simulink model "21-E"  (R2014a)
settings: Solver=FixedStepDiscrete  StartTime=0.0  StopTime=10.0  FixedStep=0.0005  RelTol=1e-3
undefined symbols (not defined in the file): add_k1_100, add_k2_100, ADDspeed, cal_acc_div, cal_acc_flo_add, cal_acc_min, cal_an_div, cal_an_min, cal_bre_div, cal_bre_en_add, cal_bre_flo_add, cal_bre_min, cal_conf_off, cal_conf_on, controller, ecucoder_acal, enres_on_add, enres_per_add
libraries: simulink x165, ec55xxlib x29
(part 1 of 6)
settings Model: Creator=ASUS  LastModifiedBy=ASUS
settings OptimizationCC: InlineParams=on  InlineInvariantSignals=on  RollThreshold=9  StateBitsets=on  DataBitsets=on  UseTempVars=on  ZeroExternalMemoryAtStartup=off  ZeroInternalMemoryAtStartup=off  EfficientFloat2IntCast=on  OptimizeModelRefInitCode=on  LifeSpan=1
settings DebuggingCC: InheritedTsInSrcMsg=none
settings HardwareCC: ProdLargestAtomicInteger=Long  ProdLargestAtomicFloat=Double  ProdIntDivRoundTo=Zero  ProdEndianess=BigEndian  ProdHWDeviceType=Freescale MPC5500
settings RTWCC: SystemTargetFile=ec55xx.tlc  MakeCommand=make_rtw optimized_fixed_point=1  GenerateMakefile=off  TemplateMakefile=ec55xx_lcc.tmf  PostCodeGenCommand=ec55xx_pst_s2(buildInfo)  Description=Target for EC55XX  GenerateReport=on  ProcessScript=ec55xx_make_rtw_hook  IncludeHyperlinkInReport=on  LaunchReport=on
settings CodeAppCC: IgnoreCustomStorageClasses=off
settings STFCustomTargetCC: ModelReferenceCompliant=off  ConcurrentExecutionCompliant=off  IncludeMdlTerminateFcn=off  GeneratePreprocessorConditionals=Use local settings  CombineOutputUpdateFcns=on  SuppressErrorStatus=on  ERTCustomFileBanners=on  SupportContinuousTime=off  SupportNonInlinedSFcns=off  MATLABClassNameForMDSCustomization=Simulink.SoftwareTarget.ERTCustomization  GRTInterface=off  SystemTargetFile=ec55xx.tlc
settings ERTTargetCC: GenerateSampleERTMain=off  ModelReferenceCompliant=off  IncludeMdlTerminateFcn=off  SuppressErrorStatus=on  GenerateASAP2=on  ERTSrcFileBannerTemplate=ec55xx_code_template.cgt  ERTHdrFileBannerTemplate=ec55xx_code_template.cgt  ERTDataSrcFileTemplate=ec55xx_code_template.cgt  ERTDataHdrFileTemplate=ec55xx_code_template.cgt  ERTCustomFileTemplate=ec55xx_file_process.tlc

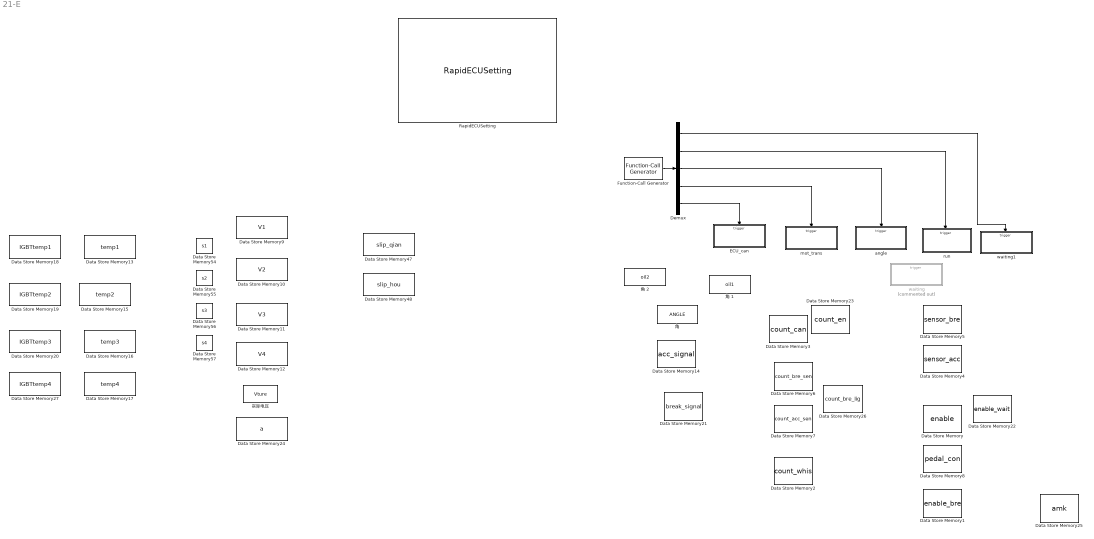
== system 21-E ==
  Data Store Memory : DataStoreMemory  DataStoreName=enable  ReadBeforeWriteMsg=warning  WriteAfterWriteMsg=warning  WriteAfterReadMsg=warning  OutDataTypeStr=boolean
  Data Store Memory1 : DataStoreMemory  DataStoreName=enable_bre  ReadBeforeWriteMsg=warning  WriteAfterWriteMsg=warning  WriteAfterReadMsg=warning  OutDataTypeStr=boolean
  Data Store Memory10 : DataStoreMemory  DataStoreName=V2  ReadBeforeWriteMsg=warning  WriteAfterWriteMsg=warning  WriteAfterReadMsg=warning  OutMin=-13000  OutMax=13000  OutDataTypeStr=double
  Data Store Memory11 : DataStoreMemory  DataStoreName=V3  ReadBeforeWriteMsg=warning  WriteAfterWriteMsg=warning  WriteAfterReadMsg=warning  OutMin=-13000  OutMax=13000  OutDataTypeStr=double
  Data Store Memory12 : DataStoreMemory  DataStoreName=V4  ReadBeforeWriteMsg=warning  WriteAfterWriteMsg=warning  WriteAfterReadMsg=warning  OutMin=-13000  OutMax=13000  OutDataTypeStr=double
  Data Store Memory13 : DataStoreMemory  DataStoreName=temp1  ReadBeforeWriteMsg=warning  WriteAfterWriteMsg=warning  WriteAfterReadMsg=warning  OutDataTypeStr=int16
  Data Store Memory14 : DataStoreMemory  DataStoreName=acc_signal  ReadBeforeWriteMsg=warning  WriteAfterWriteMsg=warning  WriteAfterReadMsg=warning  OutDataTypeStr=double
  Data Store Memory15 : DataStoreMemory  DataStoreName=temp2  ReadBeforeWriteMsg=warning  WriteAfterWriteMsg=warning  WriteAfterReadMsg=warning  OutDataTypeStr=int16
  Data Store Memory16 : DataStoreMemory  DataStoreName=temp3  ReadBeforeWriteMsg=warning  WriteAfterWriteMsg=warning  WriteAfterReadMsg=warning  OutDataTypeStr=int16
  Data Store Memory17 : DataStoreMemory  DataStoreName=temp4  ReadBeforeWriteMsg=warning  WriteAfterWriteMsg=warning  WriteAfterReadMsg=warning  OutDataTypeStr=int16
  Data Store Memory18 : DataStoreMemory  DataStoreName=IGBTtemp1  ReadBeforeWriteMsg=warning  WriteAfterWriteMsg=warning  WriteAfterReadMsg=warning  OutDataTypeStr=int16
  Data Store Memory19 : DataStoreMemory  DataStoreName=IGBTtemp2  ReadBeforeWriteMsg=warning  WriteAfterWriteMsg=warning  WriteAfterReadMsg=warning  OutDataTypeStr=int16
  Data Store Memory2 : DataStoreMemory  DataStoreName=count_whis  ReadBeforeWriteMsg=warning  WriteAfterWriteMsg=warning  WriteAfterReadMsg=warning  OutDataTypeStr=double
  Data Store Memory20 : DataStoreMemory  DataStoreName=IGBTtemp3  ReadBeforeWriteMsg=warning  WriteAfterWriteMsg=warning  WriteAfterReadMsg=warning  OutDataTypeStr=int16
  Data Store Memory21 : DataStoreMemory  DataStoreName=break_signal  ReadBeforeWriteMsg=warning  WriteAfterWriteMsg=warning  WriteAfterReadMsg=warning  OutDataTypeStr=double
  Data Store Memory22 : DataStoreMemory  DataStoreName=enable_wait  ReadBeforeWriteMsg=warning  WriteAfterWriteMsg=warning  WriteAfterReadMsg=warning  OutDataTypeStr=boolean
  Data Store Memory23 : DataStoreMemory  DataStoreName=count_en  ReadBeforeWriteMsg=warning  WriteAfterWriteMsg=warning  WriteAfterReadMsg=warning  OutDataTypeStr=double
  Data Store Memory24 : DataStoreMemory  DataStoreName=a  ReadBeforeWriteMsg=warning  WriteAfterWriteMsg=warning  WriteAfterReadMsg=warning  OutMin=-13000  OutMax=13000  OutDataTypeStr=double
  Data Store Memory25 : DataStoreMemory  DataStoreName=amk  ReadBeforeWriteMsg=warning  WriteAfterWriteMsg=warning  WriteAfterReadMsg=warning  OutDataTypeStr=uint16
  Data Store Memory26 : DataStoreMemory  DataStoreName=count_bre_lig  ReadBeforeWriteMsg=warning  WriteAfterWriteMsg=warning  WriteAfterReadMsg=warning  OutDataTypeStr=double
  Data Store Memory27 : DataStoreMemory  DataStoreName=IGBTtemp4  ReadBeforeWriteMsg=warning  WriteAfterWriteMsg=warning  WriteAfterReadMsg=warning  OutDataTypeStr=int16
  Data Store Memory3 : DataStoreMemory  DataStoreName=count_can  ReadBeforeWriteMsg=warning  WriteAfterWriteMsg=warning  WriteAfterReadMsg=warning  OutDataTypeStr=double
  Data Store Memory4 : DataStoreMemory  DataStoreName=sensor_acc  ReadBeforeWriteMsg=warning  WriteAfterWriteMsg=warning  WriteAfterReadMsg=warning  OutDataTypeStr=boolean
  Data Store Memory47 : DataStoreMemory  DataStoreName=slip_qian  ReadBeforeWriteMsg=warning  WriteAfterWriteMsg=warning  WriteAfterReadMsg=warning  OutMin=0  OutMax=1  OutDataTypeStr=double
  Data Store Memory48 : DataStoreMemory  DataStoreName=slip_hou  ReadBeforeWriteMsg=warning  WriteAfterWriteMsg=warning  WriteAfterReadMsg=warning  OutMin=0  OutMax=1  OutDataTypeStr=double
  Data Store Memory5 : DataStoreMemory  DataStoreName=sensor_bre  ReadBeforeWriteMsg=warning  WriteAfterWriteMsg=warning  WriteAfterReadMsg=warning  OutDataTypeStr=boolean
  Data Store Memory54 : DataStoreMemory  DataStoreName=s1  ReadBeforeWriteMsg=warning  WriteAfterWriteMsg=warning  WriteAfterReadMsg=warning  InitialValue=1  OutDataTypeStr=uint16
  Data Store Memory55 : DataStoreMemory  DataStoreName=s2  ReadBeforeWriteMsg=warning  WriteAfterWriteMsg=warning  WriteAfterReadMsg=warning  InitialValue=1  OutDataTypeStr=uint16
  Data Store Memory56 : DataStoreMemory  DataStoreName=s3  ReadBeforeWriteMsg=warning  WriteAfterWriteMsg=warning  WriteAfterReadMsg=warning  InitialValue=1  OutDataTypeStr=uint16
  Data Store Memory57 : DataStoreMemory  DataStoreName=s4  ReadBeforeWriteMsg=warning  WriteAfterWriteMsg=warning  WriteAfterReadMsg=warning  InitialValue=1  OutDataTypeStr=uint16
  Data Store Memory6 : DataStoreMemory  DataStoreName=count_bre_sen  ReadBeforeWriteMsg=warning  WriteAfterWriteMsg=warning  WriteAfterReadMsg=warning  OutDataTypeStr=double
  Data Store Memory7 : DataStoreMemory  DataStoreName=count_acc_sen  ReadBeforeWriteMsg=warning  WriteAfterWriteMsg=warning  WriteAfterReadMsg=warning  OutDataTypeStr=double
  Data Store Memory8 : DataStoreMemory  DataStoreName=pedal_con  ReadBeforeWriteMsg=warning  WriteAfterWriteMsg=warning  WriteAfterReadMsg=warning  OutDataTypeStr=boolean
  Data Store Memory9 : DataStoreMemory  DataStoreName=V1  ReadBeforeWriteMsg=warning  WriteAfterWriteMsg=warning  WriteAfterReadMsg=warning  OutMin=-13000  OutMax=13000  OutDataTypeStr=double
  Demux : Demux  Outputs=5
  ECU_can : Subsystem  TreatAsAtomicUnit=on
  Function-Call Generator : simulink/Ports & Subsystems/Function-Call Generator  sample_time=0.01  numberOfIterations=1
  RapidECUSetting : ec55xxlib/RapidECU_U1/RapidECUSetting
  angle : Subsystem  TreatAsAtomicUnit=on
  mot_trans : Subsystem  TreatAsAtomicUnit=on
  run : Subsystem
  waiting : Subsystem  Commented=on
  waiting1 : Subsystem
  实际电压 : DataStoreMemory  DataStoreName=Vture  ReadBeforeWriteMsg=warning  WriteAfterWriteMsg=warning  WriteAfterReadMsg=warning  OutMin=-13000  OutMax=13000  OutDataTypeStr=double
  "角 " : DataStoreMemory  DataStoreName=ANGLE  ReadBeforeWriteMsg=warning  WriteAfterWriteMsg=warning  WriteAfterReadMsg=warning  OutMin=0  OutMax=1  OutDataTypeStr=double
  角 1 : DataStoreMemory  DataStoreName=oil1  ReadBeforeWriteMsg=warning  WriteAfterWriteMsg=warning  WriteAfterReadMsg=warning  OutMin=0  OutMax=1  OutDataTypeStr=double
  角 2 : DataStoreMemory  DataStoreName=oil2  ReadBeforeWriteMsg=warning  WriteAfterWriteMsg=warning  WriteAfterReadMsg=warning  OutMin=0  OutMax=1  OutDataTypeStr=double
  wires:
  Function-Call Generator/1 -> Demux/1
  Demux/2 -> run/Trigger
  Demux/3 -> angle/Trigger
  Demux/4 -> mot_trans/Trigger
  Demux/1 -> waiting1/Trigger
  Demux/5 -> ECU_can/Trigger

== system 21-E/ECU_can ==
  note: 发送：八个温度
  note: 发送：四轮速
  note: 发送：加速线，加速角，制动油压，制动线，理想和真实侧摆速度，前轮转角，
  note: 发送：滑移率，真实和最大加速度，真实速度，
  Trigger : TriggerPort  TriggerType=function-call  PortDimensions=1
  CANTransmit1 : ec55xxlib/RapidECU_U2/07CANCommucation/CANTransmit  canmodule=B  canbuffer=8  canmessageid=hex2dec('06')  canmessagetype=Standard(11-bit ID)  datalength=8  sampletime=-1
  CANTransmit2 : ec55xxlib/RapidECU_U2/07CANCommucation/CANTransmit  canmodule=B  canbuffer=13  canmessageid=hex2dec('07')  canmessagetype=Standard(11-bit ID)  datalength=8  sampletime=-1
  CAN传输1 : ec55xxlib/RapidECU_U2/07CANCommucation/CANTransmit  canmodule=B  canbuffer=56  canmessageid=hex2dec('05')  canmessagetype=Standard(11-bit ID)  datalength=8  sampletime=-1
  CAN传输4 : ec55xxlib/RapidECU_U2/07CANCommucation/CANTransmit  canmodule=B  canbuffer=15  canmessageid=hex2dec('08')  canmessagetype=Standard(11-bit ID)  datalength=8  sampletime=-1
  Constant{2,4..9} (7 alike) : Constant  Value=100
  Data Store Read : DataStoreRead  DataStoreName=V1
  Data Store Read1 : DataStoreRead  DataStoreName=Vture
  Data Store Read10 : DataStoreRead  DataStoreName=s1
  Data Store Read11 : DataStoreRead  DataStoreName=s2
  Data Store Read12 : DataStoreRead  DataStoreName=s3
  Data Store Read13 : DataStoreRead  DataStoreName=s4
  Data Store Read14 : DataStoreRead  DataStoreName=oil1
  Data Store Read15 : DataStoreRead  DataStoreName=oil2
  Data Store Read2 : DataStoreRead  DataStoreName=ANGLE
  Data Store Read3 : DataStoreRead  DataStoreName=V2
  Data Store Read4 : DataStoreRead  DataStoreName=V3
  Data Store Read5 : DataStoreRead  DialogController=Simulink.DDGSource  DataStoreName=acc_signal
  Data Store Read6 : DataStoreRead  DataStoreName=break_signal
  Data Store Read7 : DataStoreRead  DataStoreName=V4
  Data Store Read8 : DataStoreRead  DataStoreName=slip_qian
  Data Store Read9 : DataStoreRead  DataStoreName=slip_hou
  ECU_dyn1 : Subsystem
  ECU_sig1 : Subsystem
  ECU_speed : Subsystem
  ECU_tem : Subsystem
  Gain : Gain  Gain=1e-6
  Gain1 : Gain  Gain=1e-6
  Product{,1..3} (4 alike) : Product
  Rounding Function{,1..7} (8 alike) : Rounding
  Subsystem : Subsystem
  send1_Ter{,3..5} (4 alike) : Terminator
  wires:
  ECU_tem/1(output) -> CANTransmit1/1
  Subsystem/1(tem4) -> ECU_tem/1(Mot_4_in)
  Subsystem/2(tem3) -> ECU_tem/2(Mot_3_in)
  Subsystem/3(tem2) -> ECU_tem/3(Mot_2_in)
  Subsystem/4(tem1) -> ECU_tem/4(Mot_1_in)
  Subsystem/5(IG4) -> ECU_tem/5(IGBT_4_in)
  Subsystem/6(IG3) -> ECU_tem/6(IGBT_3_in)
  Subsystem/7(IG2) -> ECU_tem/7(IGBT_2_in)
  Subsystem/8(IG1) -> ECU_tem/8(IGBT_1_in)
  Constant9/1 -> ECU_sig1/7(yaw_i_in)
  Constant8/1 -> ECU_sig1/6(yaw_r_in)
  Constant7/1 -> ECU_sig1/4(acc_a_in)
  Rounding Function1/1 -> ECU_sig1/3(bre_l_in)
  Rounding Function5/1 -> ECU_dyn1/7(speed_in)
  Rounding Function4/1 -> ECU_dyn1/5(slip_R_in)
  Rounding Function3/1 -> ECU_dyn1/6(slip_F_in)
  Rounding Function2/1 -> ECU_sig1/8(angle_in)
  Data Store Read9/1 -> Product3/2
  Constant4/1 -> Product3/1
  Product3/1 -> Rounding Function4/1
  Product2/1 -> Rounding Function3/1
  Data Store Read8/1 -> Product2/2
  Constant6/1 -> Product2/1
  Data Store Read7/1 -> ECU_speed/1(v_2R_in)
  Data Store Read4/1 -> ECU_speed/2(v_2L_in)
  Data Store Read3/1 -> ECU_speed/3(v_1R_in)
  Data Store Read/1 -> ECU_speed/4(v_1L_in)
  ECU_speed/1(output) -> CANTransmit2/1
  CANTransmit2/1 -> send1_Ter5/1  "SEND_0x07"
  CANTransmit1/1 -> send1_Ter4/1  "SEND_0x06"
  Data Store Read2/1 -> Rounding Function2/1
  Data Store Read5/1 -> Product/2
  Constant2/1 -> Product/1
  Rounding Function/1 -> ECU_sig1/5(acc_l_in)
  Product1/1 -> Rounding Function1/1
  Constant5/1 -> Product1/2
  Data Store Read6/1 -> Product1/1
  Product/1 -> Rounding Function/1
  Data Store Read1/1 -> Rounding Function5/1
  ECU_dyn1/1(output) -> CAN传输4/1
  CAN传输4/1 -> send1_Ter3/1  "SEND_0x08"
  ECU_sig1/1(output) -> CAN传输1/1
  CAN传输1/1 -> send1_Ter/1  "SEND_0x05"
  Data Store Read10/1 -> ECU_dyn1/4(s_1L_in)
  Data Store Read11/1 -> ECU_dyn1/3(s_1R_in)
  Data Store Read12/1 -> ECU_dyn1/2(s_2L_in)
  Data Store Read13/1 -> ECU_dyn1/1(s_2R_in)
  Data Store Read14/1 -> Gain1/1
  Data Store Read15/1 -> Gain/1
  Gain/1 -> Rounding Function7/1
  Gain1/1 -> Rounding Function6/1
  Rounding Function6/1 -> ECU_sig1/2(bre_o_1_in)
  Rounding Function7/1 -> ECU_sig1/1(bre_o_2_in)

== system 21-E/angle ==
  note: 接收：转角,角速度，最大角速度
  note: 接收：转角,角速度，最大角速度
  Trigger : TriggerPort  TriggerType=function-call  PortDimensions=1
  CAN接收1 : ec55xxlib/RapidECU_U2/07CANCommucation/CANReceive  canmodule=B  canbuffer=16  canmessageid=hex2dec('0001')  canmessagetype=Standard(11-bit ID)  datalength=8  sampletime=-1
  Constant : Constant  Value=2780
  Constant1 : Constant  Value=31
  ECCalVar : Constant  InitFcn=ecucoder_acal;  Value=cal_an_min  OutDataTypeStr=Inherit: Inherit via back propagation  SampleTime=-1
  ECCalVar2 : Constant  InitFcn=ecucoder_acal;  Value=cal_an_div  OutDataTypeStr=Inherit: Inherit via back propagation  SampleTime=-1
  Product1 : Product  Inputs=*/
  Sum : Sum  Inputs=|+-
  Sum1 : Sum  Inputs=|++
  Sum2 : Sum  Inputs=|++
  Terminator{,1..7} (8 alike) : Terminator
  angle2 : Subsystem
  模数转换 : DataTypeConversion  OutDataTypeStr=double
  模数转换1 : DataTypeConversion  OutDataTypeStr=double
  "角 " : DataStoreWrite  DataStoreName=ANGLE
  wires:
  Constant/1 -> Sum1/1
  ECCalVar/1 -> Sum1/2
  Sum/1 -> Product1/1  "calan_min"
  Product1/1 -> "角 "/1  "cal_an"
  Constant1/1 -> Sum2/1
  ECCalVar2/1 -> Sum2/2
  angle2/4(angle_2_Out) -> 模数转换/1  "angle01_2"
  angle2/5(angle_1_Out) -> 模数转换1/1  "angle01_1"
  模数转换/1 -> Terminator/1  "an01_2"
  模数转换1/1 -> Terminator1/1  "an01_1"
  angle2/3(un_1_Out) -> Terminator4/1
  angle2/2(un_2_Out) -> Terminator3/1  "un6"
  angle2/1(un_3_Out) -> Terminator2/1  "un1"
  CAN接收1/5 -> Terminator6/1
  CAN接收1/1 -> angle2/Trigger
  CAN接收1/4 -> angle2/1(input)
  CAN接收1/3 -> Terminator7/1
  CAN接收1/2 -> Terminator5/1  "ooo1"

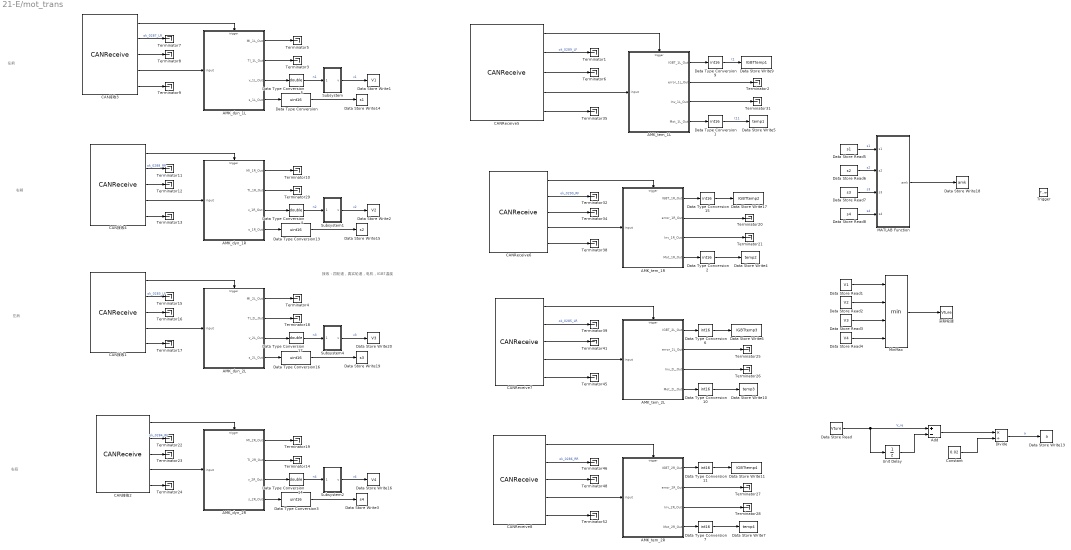
== system 21-E/mot_trans ==
  note: 接收：四轮速，真实轮速，电机，IGBT温度
  note: 右后
  note: 左后
  note: 右前
  note: 左前
  Trigger : TriggerPort  TriggerType=function-call  PortDimensions=1
  AMK_dyn_1L : Subsystem
  AMK_dyn_1R : Subsystem
  AMK_dyn_2L : Subsystem
  AMK_dyn_2R : Subsystem
  AMK_tem_1L : Subsystem
  AMK_tem_1R : Subsystem
  AMK_tem_2L : Subsystem
  AMK_tem_2R : Subsystem
  Add : Sum  Inputs=+-
  CANReceive5 : ec55xxlib/RapidECU_U2/07CANCommucation/CANReceive  canmodule=A  canbuffer=4  canmessageid=hex2dec('0289')  canmessagetype=Standard(11-bit ID)  datalength=8  sampletime=-1
  CANReceive6 : ec55xxlib/RapidECU_U2/07CANCommucation/CANReceive  canmodule=A  canbuffer=5  canmessageid=hex2dec('0290')  canmessagetype=Standard(11-bit ID)  datalength=8  sampletime=-1
  CANReceive7 : ec55xxlib/RapidECU_U2/07CANCommucation/CANReceive  canmodule=A  canbuffer=6  canmessageid=hex2dec('0285')  canmessagetype=Standard(11-bit ID)  datalength=8  sampletime=-1
  CANReceive8 : ec55xxlib/RapidECU_U2/07CANCommucation/CANReceive  canmodule=A  canbuffer=7  canmessageid=hex2dec('0286')  canmessagetype=Standard(11-bit ID)  datalength=8  sampletime=-1
  CAN接收1 : ec55xxlib/RapidECU_U2/07CANCommucation/CANReceive  canmodule=A  canbuffer=0  canmessageid=hex2dec('0283')  canmessagetype=Standard(11-bit ID)  datalength=8  sampletime=-1
  CAN接收2 : ec55xxlib/RapidECU_U2/07CANCommucation/CANReceive  canmodule=A  canbuffer=1  canmessageid=hex2dec('284')  canmessagetype=Standard(11-bit ID)  datalength=8  sampletime=-1
  CAN接收3 : ec55xxlib/RapidECU_U2/07CANCommucation/CANReceive  canmodule=A  canbuffer=2  canmessageid=hex2dec('0287')  canmessagetype=Standard(11-bit ID)  datalength=8  sampletime=-1
  CAN接收4 : ec55xxlib/RapidECU_U2/07CANCommucation/CANReceive  canmodule=A  canbuffer=3  canmessageid=hex2dec('0288')  canmessagetype=Standard(11-bit ID)  datalength=8  sampletime=-1
  Constant : Constant  Value=0.02
  Data Store Read : DataStoreRead  DataStoreName=Vture
  Data Store Read1 : DataStoreRead  DataStoreName=V1
  Data Store Read2 : DataStoreRead  DataStoreName=V2
  Data Store Read3 : DataStoreRead  DataStoreName=V3
  Data Store Read4 : DataStoreRead  DataStoreName=V4
  Data Store Read5 : DataStoreRead  DataStoreName=s1
  Data Store Read6 : DataStoreRead  DataStoreName=s2
  Data Store Read7 : DataStoreRead  DataStoreName=s3
  Data Store Read8 : DataStoreRead  DataStoreName=s4
  Data Store Write1 : DataStoreWrite  DataStoreName=V1
  Data Store Write10 : DataStoreWrite  DataStoreName=temp3
  Data Store Write11 : DataStoreWrite  DataStoreName=IGBTtemp4
  Data Store Write13 : DataStoreWrite  DataStoreName=a
  Data Store Write14 : DataStoreWrite  DataStoreName=s1
  Data Store Write15 : DataStoreWrite  DataStoreName=s2
  Data Store Write16 : DataStoreWrite  DataStoreName=V4
  Data Store Write17 : DataStoreWrite  DataStoreName=IGBTtemp2
  Data Store Write18 : DataStoreWrite  DataStoreName=amk
  Data Store Write19 : DataStoreWrite  DataStoreName=s3
  Data Store Write2 : DataStoreWrite  DataStoreName=V2
  Data Store Write20 : DataStoreWrite  DataStoreName=V3
  Data Store Write3 : DataStoreWrite  DataStoreName=s4
  Data Store Write4 : DataStoreWrite  DataStoreName=temp2
  Data Store Write5 : DataStoreWrite  DataStoreName=temp1
  Data Store Write6 : DataStoreWrite  DataStoreName=IGBTtemp3
  Data Store Write7 : DataStoreWrite  DataStoreName=temp4
  Data Store Write9 : DataStoreWrite  DialogController=Simulink.DDGSource  DataStoreName=IGBTtemp1
  Data Type Conversion{,3,13,16} (4 alike) : DataTypeConversion  OutDataTypeStr=uint16
  Data Type Conversion{1..2,6..7,9..11,15} (8 alike) : DataTypeConversion  OutDataTypeStr=int16
  Data Type Conversion{4..5,14,17} (4 alike) : DataTypeConversion  OutDataTypeStr=double
  Divide : Product  Inputs=*/
  MATLAB Function : MATLAB Function  TreatAsAtomicUnit=on
  MinMax : MinMax  Inputs=4
  Subsystem : Subsystem
  Subsystem1 : Subsystem
  Subsystem2 : Subsystem
  Subsystem4 : Subsystem
  Terminator{1..29,31..32,34..35,38..39,41,45..46,48,52} (40 alike) : Terminator
  Unit Delay : UnitDelay  SampleTime=-1
  "实际轮速 " : DataStoreWrite  DialogController=Simulink.DDGSource  DataStoreName=Vture
  wires:
  AMK_dyn_1L/2(TI_1L_Out) -> Terminator3/1
  MinMax/1 -> "实际轮速 "/1
  Data Type Conversion4/1 -> Subsystem1/1(ome)  "n2"
  Data Type Conversion5/1 -> Subsystem/1(ome)  "n1"
  CANReceive5/1 -> AMK_tem_1L/Trigger
  CANReceive5/2 -> Terminator1/1  "ok_0289_LF"
  CANReceive5/4 -> AMK_tem_1L/1(input)
  CANReceive5/3 -> Terminator6/1
  CANReceive5/5 -> Terminator35/1
  CANReceive6/1 -> AMK_tem_1R/Trigger
  CANReceive6/2 -> Terminator32/1  "ok_0290_RF"
  CANReceive6/4 -> AMK_tem_1R/1(input)
  CANReceive6/3 -> Terminator34/1
  CANReceive6/5 -> Terminator38/1
  CANReceive7/2 -> Terminator39/1  "ok_0285_LR"
  CANReceive7/4 -> AMK_tem_2L/1(input)
  CANReceive7/3 -> Terminator41/1
  CANReceive7/5 -> Terminator45/1
  CANReceive8/1 -> AMK_tem_2R/Trigger
  CANReceive8/2 -> Terminator46/1  "ok_0286_RR"
  CANReceive8/4 -> AMK_tem_2R/1(input)
  CANReceive8/3 -> Terminator48/1
  CANReceive8/5 -> Terminator52/1
  Data Type Conversion1/1 -> Data Store Write5/1  "t11"
  Data Type Conversion9/1 -> Data Store Write9/1  "t1"
  Subsystem/1(v) -> Data Store Write1/1  "v1"
  Subsystem1/1(v) -> Data Store Write2/1  "v2"
  Data Store Read/1 -> Unit Delay/1, Add/1  "V_re"
  Unit Delay/1 -> Add/2
  Add/1 -> Divide/1
  Constant/1 -> Divide/2
  Divide/1 -> Data Store Write13/1  "a"
  Data Type Conversion/1 -> Data Store Write14/1
  Data Type Conversion13/1 -> Data Store Write15/1
  Data Store Read5/1 -> MATLAB Function/1(s1)  "s1"
  Data Store Read6/1 -> MATLAB Function/2(s2)  "s2"
  Data Store Read7/1 -> MATLAB Function/3(s3)  "s3"
  Data Store Read8/1 -> MATLAB Function/4(s4)  "s4"
  AMK_dyn_1L/3(v_1L_Out) -> Data Type Conversion5/1
  AMK_dyn_1L/4(s_1L_Out) -> Data Type Conversion/1
  AMK_dyn_1L/1(MI_1L_Out) -> Terminator5/1
  AMK_dyn_1R/4(s_1R_Out) -> Data Type Conversion13/1
  AMK_dyn_1R/3(v_1R_Out) -> Data Type Conversion4/1
  AMK_dyn_1R/2(TI_1R_Out) -> Terminator29/1
  AMK_dyn_1R/1(MI_1R_Out) -> Terminator10/1
  Data Type Conversion17/1 -> Subsystem4/1(ome)  "n3"
  Subsystem4/1(v) -> Data Store Write20/1  "v3"
  Data Type Conversion16/1 -> Data Store Write19/1
  AMK_dyn_2L/4(s_2L_Out) -> Data Type Conversion16/1
  AMK_dyn_2L/2(TI_2L_Out) -> Terminator18/1
  AMK_dyn_2L/1(MI_2L_Out) -> Terminator4/1
  AMK_dyn_2L/3(v_2L_Out) -> Data Type Conversion17/1
  Data Type Conversion14/1 -> Subsystem2/1(ome)  "n4"
  Subsystem2/1(v) -> Data Store Write16/1  "v4"
  Data Type Conversion3/1 -> Data Store Write3/1
  AMK_dyn_2R/4(s_2R_Out) -> Data Type Conversion3/1
  AMK_dyn_2R/2(TI_2R_Out) -> Terminator14/1
  AMK_dyn_2R/1(MI_2R_Out) -> Terminator19/1
  AMK_dyn_2R/3(v_2R_Out) -> Data Type Conversion14/1
  Data Store Read4/1 -> MinMax/4
  Data Store Read3/1 -> MinMax/3
  Data Store Read2/1 -> MinMax/2
  Data Store Read1/1 -> MinMax/1
  AMK_tem_1L/1(IGBT_1L_Out) -> Data Type Conversion9/1
  AMK_tem_1L/2(error_1L_Out) -> Terminator2/1
  AMK_tem_1L/4(Mot_1L_Out) -> Data Type Conversion1/1
  AMK_tem_1L/3(Inv_1L_Out) -> Terminator31/1
  Data Type Conversion2/1 -> Data Store Write4/1
  Data Type Conversion15/1 -> Data Store Write17/1
  AMK_tem_1R/1(IGBT_1R_Out) -> Data Type Conversion15/1
  AMK_tem_1R/2(error_1R_Out) -> Terminator20/1
  AMK_tem_1R/4(Mot_1R_Out) -> Data Type Conversion2/1
  AMK_tem_1R/3(Inv_1R_Out) -> Terminator21/1
  Data Type Conversion10/1 -> Data Store Write10/1
  Data Type Conversion6/1 -> Data Store Write6/1
  AMK_tem_2L/1(IGBT_2L_Out) -> Data Type Conversion6/1
  AMK_tem_2L/2(error_2L_Out) -> Terminator25/1
  AMK_tem_2L/4(Mot_2L_Out) -> Data Type Conversion10/1
  AMK_tem_2L/3(Inv_2L_Out) -> Terminator26/1
  CANReceive7/1 -> AMK_tem_2L/Trigger
  Data Type Conversion7/1 -> Data Store Write7/1
  Data Type Conversion11/1 -> Data Store Write11/1
  AMK_tem_2R/1(IGBT_2R_Out) -> Data Type Conversion11/1
  AMK_tem_2R/2(error_2R_Out) -> Terminator27/1
  AMK_tem_2R/4(Mot_2R_Out) -> Data Type Conversion7/1
  AMK_tem_2R/3(Inv_2R_Out) -> Terminator28/1
  MATLAB Function/1(amk) -> Data Store Write18/1
  CAN接收3/4 -> AMK_dyn_1L/1(input)
  CAN接收3/1 -> AMK_dyn_1L/Trigger
  CAN接收3/2 -> Terminator7/1  "ok_0287_LR"
  CAN接收3/3 -> Terminator8/1
  CAN接收3/5 -> Terminator9/1
  CAN接收4/5 -> Terminator13/1
  CAN接收4/3 -> Terminator12/1
  CAN接收4/2 -> Terminator11/1  "ok_0288_RR"
  CAN接收4/4 -> AMK_dyn_1R/1(input)
  CAN接收4/1 -> AMK_dyn_1R/Trigger
  CAN接收1/5 -> Terminator17/1
  CAN接收1/3 -> Terminator16/1
  CAN接收1/2 -> Terminator15/1  "ok_0283_LF"
  CAN接收1/4 -> AMK_dyn_2L/1(input)
  CAN接收1/1 -> AMK_dyn_2L/Trigger
  CAN接收2/5 -> Terminator24/1
  CAN接收2/4 -> AMK_dyn_2R/1(input)
  CAN接收2/3 -> Terminator23/1
  CAN接收2/2 -> Terminator22/1  "ok_0284_RF"
  CAN接收2/1 -> AMK_dyn_2R/Trigger

== system 21-E/run ==
  Trigger : TriggerPort  TriggerType=function-call  PortDimensions=1
  Subsystem : Subsystem
  analog_acq : Subsystem
  cal&con : Subsystem
  ctrl : Subsystem
  emp : Subsystem
  wires:
  analog_acq/1(acc_ana) -> cal&con/1(acc_ana)
  emp/2(acc_fin) -> ctrl/2(acc)
  analog_acq/2(bre_ana) -> cal&con/2(bre_ana)
  cal&con/1(acc) -> emp/1(acc)
  cal&con/2(bre) -> emp/2(bre)
  analog_acq/3(oilpre1) -> Subsystem/2("pressure sensor_front（pa） ")
  analog_acq/4(oilpre2) -> Subsystem/3("pressure sensor_rear（pa） ")
  emp/1(bre_fin) -> Subsystem/1(bra signal), ctrl/1(bre)
  Subsystem/1("FL motor Torque ") -> ctrl/3(TN1L)
  Subsystem/4(RR motor Torque1) -> ctrl/6(TN2R)
  Subsystem/2(FR motor Torque) -> ctrl/4(TN1R)
  Subsystem/3(RL motor Torque) -> ctrl/5(TN2L)

== system 21-E/waiting ==
  Trigger : TriggerPort  TriggerType=function-call  PortDimensions=1
  AnalogInput : ec55xxlib/RapidECU_U1/02AnalogInput/AnalogInput  channel=16: I_AN05_28V  sampletime=-1
  Constant : Constant  Value=20000  OutDataTypeStr=uint16
  Constant1 : Constant  Value=0
  Constant6 : Constant  Value=256
  Constant7 : Constant  Value=30976
  Data Store Read{,2,4,7} (4 alike) : DataStoreRead  Priority=0  DialogController=Simulink.DDGSource  DataStoreName=enable
  Data Store Read1 : DataStoreRead  Priority=0  DialogController=Simulink.DDGSource  DataStoreName=enable_bre
  Data Store Read10 : DataStoreRead  Priority=0  DataStoreName=enable_wait
  Data Store Read11 : DataStoreRead  Priority=0  DialogController=Simulink.DDGSource  DataStoreName=count_en
  Data Store Read3 : DataStoreRead  Priority=0  DataStoreName=enable_bre
  Data Store Read5 : DataStoreRead  Priority=0  DataStoreName=amk
  Data Store Read6 : DataStoreRead  Priority=0  DataStoreName=amk
  Data Store Read8 : DataStoreRead  DataStoreName=enable_wait
  Data Store Read9 : DataStoreRead  Priority=1  DataStoreName=enable_wait
  Data Store Write : DataStoreWrite  DataStoreName=enable_wait
  Data Store Write1 : DataStoreWrite  DialogController=Simulink.DDGSource  DataStoreName=enable
  Data Store Write2 : DataStoreWrite  Priority=1  DataStoreName=enable_wait
  Data Store Write3 : DataStoreWrite  Commented=on  DialogController=Simulink.DDGSource  DataStoreName=enable
  Data Type Conversion : DataTypeConversion  OutDataTypeStr=uint32
  Data Type Conversion1 : DataTypeConversion  OutDataTypeStr=uint32
  Logical Operator : Logic  Inputs=4  AllPortsSameDT=off  OutDataTypeStr=boolean
  Logical Operator1 : Logic  Operator=NOT  AllPortsSameDT=off  OutDataTypeStr=boolean
  Logical Operator2 : Logic  Commented=on  AllPortsSameDT=off  OutDataTypeStr=boolean
  MATLAB Function : MATLAB Function  TreatAsAtomicUnit=on
  MATLAB Function1 : MATLAB Function  TreatAsAtomicUnit=on
  MATLAB Function2 : MATLAB Function  Commented=on  TreatAsAtomicUnit=on
  MATLAB Function3 : MATLAB Function  TreatAsAtomicUnit=on
  MATLAB Function4 : MATLAB Function  Commented=on  TreatAsAtomicUnit=on
  MATLAB Function5 : MATLAB Function  TreatAsAtomicUnit=on
  Relational Operator : RelationalOperator  OutDataTypeStr=boolean
  Relational Operator1 : RelationalOperator  Operator===  OutDataTypeStr=boolean
  Relational Operator2 : RelationalOperator  Operator=~=  OutDataTypeStr=boolean
  Relational Operator3 : RelationalOperator  Operator===  OutDataTypeStr=boolean
  Subsystem : Subsystem
  Terminator : Terminator
  en_lig : ec55xxlib/RapidECU_U1/06PowerDriverPWM/PowerDriverPWM  channel=117: O_PWM11_HS2A9  sampletime=-1
  wires:
  Constant6/1 -> Relational Operator3/2
  Data Store Read6/1 -> Relational Operator3/1
  Constant7/1 -> Relational Operator2/2
  Data Store Read5/1 -> Relational Operator2/1
  Data Store Read9/1 -> MATLAB Function5/2(wait), Subsystem/1(wait), MATLAB Function/1(u)  "wait"
  MATLAB Function3/1(y) -> Data Store Write/1  "tri_wait"
  Logical Operator/1 -> MATLAB Function3/1(u)
  Relational Operator/1 -> Logical Operator/1, Logical Operator2/1
  Logical Operator1/1 -> Logical Operator2/2
  Data Store Read3/1 -> Logical Operator1/1
  Constant/1 -> Relational Operator/2
  Relational Operator1/1 -> Logical Operator/2
  Data Store Read/1 -> Relational Operator1/2  "enable"
  Constant1/1 -> Relational Operator1/1
  Logical Operator2/1 -> MATLAB Function2/1(u)
  AnalogInput/1 -> Relational Operator/1  "en_vol"
  Data Store Read1/1 -> Logical Operator/3
  Data Store Read7/1 -> MATLAB Function/2(en)
  Data Store Read8/1 -> MATLAB Function3/2(wait)
  MATLAB Function/1(y) -> Data Store Write1/1
  MATLAB Function1/1(y) -> Data Store Write2/1
  Data Store Read10/1 -> MATLAB Function1/2(wait)
  MATLAB Function4/1(y) -> Data Store Write3/1
  Data Store Read2/1 -> MATLAB Function5/1(en), MATLAB Function1/1(en)
  MATLAB Function5/1(p) -> Data Type Conversion/1
  MATLAB Function5/2(o) -> Data Type Conversion1/1
  Data Type Conversion/1 -> en_lig/1
  Data Type Conversion1/1 -> en_lig/2
  Relational Operator3/1 -> Logical Operator/4
  Data Store Read11/1 -> Terminator/1  "count"

== system 21-E/waiting1 ==
  Trigger : TriggerPort  TriggerType=function-call  PortDimensions=1
  AnalogInput : ec55xxlib/RapidECU_U1/02AnalogInput/AnalogInput  channel=16: I_AN05_28V  sampletime=-1
  Constant : Constant  Value=20000  OutDataTypeStr=uint16
  Constant1 : Constant  Value=0
  Constant2 : Constant  Value=30976
  Constant3 : Constant
  Constant6 : Constant  Value=256
  Constant7 : Constant  Value=30976
  Data Store Read : DataStoreRead  Priority=0  DialogController=Simulink.DDGSource  DataStoreName=enable
  Data Store Read1 : DataStoreRead  Priority=0  DialogController=Simulink.DDGSource  DataStoreName=enable_bre
  Data Store Read10 : DataStoreRead  Priority=0  DataStoreName=enable_wait
  Data Store Read11 : DataStoreRead  Priority=1  DataStoreName=count_en
  Data Store Read12 : DataStoreRead  Priority=0  DataStoreName=amk
  Data Store Read2 : DataStoreRead  Priority=0  DialogController=Simulink.DDGSource  DataStoreName=enable
  Data Store Read3 : DataStoreRead  Priority=0  DataStoreName=enable_bre
  Data Store Read4 : DataStoreRead  Priority=0  Commented=on  DialogController=Simulink.DDGSource  DataStoreName=enable
  Data Store Read5 : DataStoreRead  Priority=0  DataStoreName=amk
  Data Store Read6 : DataStoreRead  Priority=0  DataStoreName=amk
  Data Store Read7 : DataStoreRead  Priority=0  DialogController=Simulink.DDGSource  DataStoreName=enable
  Data Store Read8 : DataStoreRead  DataStoreName=enable_wait
  Data Store Read9 : DataStoreRead  Priority=1  DataStoreName=enable_wait
  Data Store Write : DataStoreWrite  DataStoreName=enable_wait
  Data Store Write1 : DataStoreWrite  DialogController=Simulink.DDGSource  DataStoreName=enable
  Data Store Write2 : DataStoreWrite  Priority=1  DataStoreName=enable_wait
  Data Store Write3 : DataStoreWrite  Commented=on  DialogController=Simulink.DDGSource  DataStoreName=enable
  Data Store Write4 : DataStoreWrite  DialogController=Simulink.DDGSource  DataStoreName=enable
  Data Type Conversion : DataTypeConversion  OutDataTypeStr=uint32
  Data Type Conversion1 : DataTypeConversion  OutDataTypeStr=uint32
  Logical Operator : Logic  Inputs=4  AllPortsSameDT=off  OutDataTypeStr=boolean
  Logical Operator1 : Logic  Operator=NOT  AllPortsSameDT=off  OutDataTypeStr=boolean
  Logical Operator2 : Logic  AllPortsSameDT=off  OutDataTypeStr=boolean
  Logical Operator3 : Logic  Operator=OR  AllPortsSameDT=off  OutDataTypeStr=boolean
  Logical Operator4 : Logic  AllPortsSameDT=off  OutDataTypeStr=boolean
  Logical Operator5 : Logic  Operator=NOT  AllPortsSameDT=off  OutDataTypeStr=boolean
  MATLAB Function : MATLAB Function  TreatAsAtomicUnit=on
  MATLAB Function1 : MATLAB Function  TreatAsAtomicUnit=on
  MATLAB Function2 : MATLAB Function  TreatAsAtomicUnit=on
  MATLAB Function3 : MATLAB Function  TreatAsAtomicUnit=on
  MATLAB Function4 : MATLAB Function  Commented=on  TreatAsAtomicUnit=on
  MATLAB Function5 : MATLAB Function  TreatAsAtomicUnit=on
  Relational Operator : RelationalOperator  OutDataTypeStr=boolean
  Relational Operator1 : RelationalOperator  Operator===  OutDataTypeStr=boolean
  Relational Operator2 : RelationalOperator  Operator=~=  OutDataTypeStr=boolean
  Relational Operator3 : RelationalOperator  Operator===  OutDataTypeStr=boolean
  Relational Operator4 : RelationalOperator  Operator===  OutDataTypeStr=boolean
  Subsystem : Subsystem
  Terminator : Terminator
  en_lig : ec55xxlib/RapidECU_U1/06PowerDriverPWM/PowerDriverPWM  channel=117: O_PWM11_HS2A9  sampletime=-1
  wires:
  Logical Operator3/1 -> Logical Operator5/1
  Logical Operator4/1 -> Data Store Write4/1
  Relational Operator4/1 -> Logical Operator4/1
  Data Store Read12/1 -> Relational Operator4/1
  Constant2/1 -> Relational Operator4/2
  Data Store Read5/1 -> Relational Operator2/1  "amk"
  Data Store Read11/1 -> Terminator/1  "count"
  Relational Operator2/1 -> Logical Operator3/2
  Relational Operator3/1 -> Logical Operator/4
  Data Type Conversion1/1 -> en_lig/2
  Data Type Conversion/1 -> en_lig/1
  MATLAB Function5/2(o) -> Data Type Conversion1/1
  MATLAB Function5/1(p) -> Data Type Conversion/1
  Data Store Read2/1 -> MATLAB Function1/1(en), MATLAB Function5/1(en)
  MATLAB Function4/1(y) -> Data Store Write3/1
  Data Store Read4/1 -> MATLAB Function4/2(en)
  Data Store Read10/1 -> MATLAB Function1/2(wait)
  MATLAB Function1/1(y) -> Data Store Write2/1
  MATLAB Function/1(y) -> Data Store Write1/1
  Data Store Read8/1 -> MATLAB Function3/2(wait)
  Data Store Read7/1 -> MATLAB Function/2(en)
  Data Store Read1/1 -> Logical Operator/3
  AnalogInput/1 -> Relational Operator/1  "en_vol"
  Logical Operator2/1 -> MATLAB Function2/1(u)
  Constant1/1 -> Relational Operator1/1
  Data Store Read/1 -> Relational Operator1/2  "enable"
  Relational Operator1/1 -> Logical Operator/2
  Constant/1 -> Relational Operator/2
  Data Store Read3/1 -> Logical Operator1/1
  Logical Operator1/1 -> Logical Operator2/2
  Relational Operator/1 -> Logical Operator2/1, Logical Operator/1
  Logical Operator/1 -> MATLAB Function3/1(u)
  MATLAB Function3/1(y) -> Data Store Write/1  "tri_wait"
  Data Store Read9/1 -> MATLAB Function/1(u), Subsystem/1(wait), MATLAB Function5/2(wait)  "wait"
  MATLAB Function2/1(y) -> Logical Operator3/1
  Constant7/1 -> Relational Operator2/2
  Data Store Read6/1 -> Relational Operator3/1
  Constant6/1 -> Relational Operator3/2
  Constant3/1 -> Logical Operator4/2

== system 21-E/ECU_can/ECU_dyn1 ==
  s_2R_in : Inport
  s_2L_in : Inport  Port=2
  s_1R_in : Inport  Port=3
  s_1L_in : Inport  Port=4
  slip_R_in : Inport  Port=5
  slip_F_in : Inport  Port=6
  speed_in : Inport  Port=7
  Conv{1..8} (8 alike) : DataTypeConversion
  ECU_dyn_DLC : Constant  Value=8  OutDataTypeStr=uint8
  ECU_dyn_DLC_Out : Terminator
  ECU_dyn_ID : Constant  Value=8  OutDataTypeStr=single
  ECU_dyn_ID_Out : Terminator
  ECU_dyn_mux : Mux  Inputs=8
  or{1..8} (8 alike) : simulink/Logic and Bit Operations/Bitwise Operator  logicop=OR  UseBitMask=off  NumInputPorts=7  BitMask=bin2dec('11011001')  BitMaskRealWorld=Stored Integer
  s_1L : Subsystem
  s_1R : Subsystem
  s_2L : Subsystem
  s_2R : Subsystem
  slip_F : Subsystem
  slip_R : Subsystem
  speed : Subsystem
  output : Outport
  wires:
  speed_in/1 -> speed/1(speed)
  slip_F_in/1 -> slip_F/1(slip_F)
  slip_R_in/1 -> slip_R/1(slip_R)
  s_1L_in/1 -> s_1L/1(s_1L)
  s_1R_in/1 -> s_1R/1(s_1R)
  s_2L_in/1 -> s_2L/1(s_2L)
  s_2R_in/1 -> s_2R/1(s_2R)
  ECU_dyn_DLC/1 -> ECU_dyn_DLC_Out/1
  ECU_dyn_ID/1 -> ECU_dyn_ID_Out/1
  Conv8/1 -> ECU_dyn_mux/8
  or8/1 -> Conv8/1
  Conv7/1 -> ECU_dyn_mux/7
  or7/1 -> Conv7/1
  Conv6/1 -> ECU_dyn_mux/6
  or6/1 -> Conv6/1
  Conv5/1 -> ECU_dyn_mux/5
  or5/1 -> Conv5/1
  Conv4/1 -> ECU_dyn_mux/4
  or4/1 -> Conv4/1
  Conv3/1 -> ECU_dyn_mux/3
  or3/1 -> Conv3/1
  Conv2/1 -> ECU_dyn_mux/2
  or2/1 -> Conv2/1
  Conv1/1 -> ECU_dyn_mux/1
  or1/1 -> Conv1/1
  speed/8(output8) -> or8/7
  speed/7(output7) -> or7/7
  speed/6(output6) -> or6/7
  speed/5(output5) -> or5/7
  speed/4(output4) -> or4/7
  speed/3(output3) -> or3/7
  speed/2(output2) -> or2/7
  speed/1(output1) -> or1/7
  slip_F/8(output8) -> or8/6
  slip_F/7(output7) -> or7/6
  slip_F/6(output6) -> or6/6
  slip_F/5(output5) -> or5/6
  slip_F/4(output4) -> or4/6
  slip_F/3(output3) -> or3/6
  slip_F/2(output2) -> or2/6
  slip_F/1(output1) -> or1/6
  slip_R/8(output8) -> or8/5
  slip_R/7(output7) -> or7/5
  slip_R/6(output6) -> or6/5
  slip_R/5(output5) -> or5/5
  slip_R/4(output4) -> or4/5
  slip_R/3(output3) -> or3/5
  slip_R/2(output2) -> or2/5
  slip_R/1(output1) -> or1/5
  s_1L/8(output8) -> or8/4
  s_1L/7(output7) -> or7/4
  s_1L/6(output6) -> or6/4
  s_1L/5(output5) -> or5/4
  s_1L/4(output4) -> or4/4
  s_1L/3(output3) -> or3/4
  s_1L/2(output2) -> or2/4
  s_1L/1(output1) -> or1/4
  s_1R/8(output8) -> or8/3
  s_1R/7(output7) -> or7/3
  s_1R/6(output6) -> or6/3
  s_1R/5(output5) -> or5/3
  s_1R/4(output4) -> or4/3
  s_1R/3(output3) -> or3/3
  s_1R/2(output2) -> or2/3
  s_1R/1(output1) -> or1/3
  s_2L/8(output8) -> or8/2
  s_2L/7(output7) -> or7/2
  s_2L/6(output6) -> or6/2
  s_2L/5(output5) -> or5/2
  s_2L/4(output4) -> or4/2
  s_2L/3(output3) -> or3/2
  s_2L/2(output2) -> or2/2
  s_2L/1(output1) -> or1/2
  s_2R/8(output8) -> or8/1
  s_2R/7(output7) -> or7/1
  s_2R/6(output6) -> or6/1
  s_2R/5(output5) -> or5/1
  s_2R/4(output4) -> or4/1
  s_2R/3(output3) -> or3/1
  s_2R/2(output2) -> or2/1
  s_2R/1(output1) -> or1/1
  ECU_dyn_mux/1 -> output/1

== system 21-E/ECU_can/ECU_sig1 ==
  bre_o_2_in : Inport
  bre_o_1_in : Inport  Port=2
  bre_l_in : Inport  Port=3
  acc_a_in : Inport  Port=4
  acc_l_in : Inport  Port=5
  yaw_r_in : Inport  Port=6
  yaw_i_in : Inport  Port=7
  angle_in : Inport  Port=8
  Conv{1..8} (8 alike) : DataTypeConversion
  ECU_sig_DLC : Constant  Value=8  OutDataTypeStr=uint8
  ECU_sig_DLC_Out : Terminator
  ECU_sig_ID : Constant  Value=5  OutDataTypeStr=single
  ECU_sig_ID_Out : Terminator
  ECU_sig_mux : Mux  Inputs=8
  acc_a : Subsystem
  acc_l : Subsystem
  angle : Subsystem
  bre_l : Subsystem
  bre_o_1 : Subsystem
  bre_o_2 : Subsystem
  or{1..8} (8 alike) : simulink/Logic and Bit Operations/Bitwise Operator  logicop=OR  UseBitMask=off  NumInputPorts=8  BitMask=bin2dec('11011001')  BitMaskRealWorld=Stored Integer
  yaw_i : Subsystem
  yaw_r : Subsystem
  output : Outport
  wires:
  angle_in/1 -> angle/1(angle)
  yaw_i_in/1 -> yaw_i/1(yaw_i)
  yaw_r_in/1 -> yaw_r/1(yaw_r)
  acc_l_in/1 -> acc_l/1(acc_l)
  acc_a_in/1 -> acc_a/1(acc_a)
  bre_l_in/1 -> bre_l/1(bre_l)
  bre_o_1_in/1 -> bre_o_1/1(bre_o_1)
  bre_o_2_in/1 -> bre_o_2/1(bre_o_2)
  ECU_sig_DLC/1 -> ECU_sig_DLC_Out/1
  ECU_sig_ID/1 -> ECU_sig_ID_Out/1
  Conv8/1 -> ECU_sig_mux/8
  or8/1 -> Conv8/1
  Conv7/1 -> ECU_sig_mux/7
  or7/1 -> Conv7/1
  Conv6/1 -> ECU_sig_mux/6
  or6/1 -> Conv6/1
  Conv5/1 -> ECU_sig_mux/5
  or5/1 -> Conv5/1
  Conv4/1 -> ECU_sig_mux/4
  or4/1 -> Conv4/1
  Conv3/1 -> ECU_sig_mux/3
  or3/1 -> Conv3/1
  Conv2/1 -> ECU_sig_mux/2
  or2/1 -> Conv2/1
  Conv1/1 -> ECU_sig_mux/1
  or1/1 -> Conv1/1
  angle/8(output8) -> or8/8
  angle/7(output7) -> or7/8
  angle/6(output6) -> or6/8
  angle/5(output5) -> or5/8
  angle/4(output4) -> or4/8
  angle/3(output3) -> or3/8
  angle/2(output2) -> or2/8
  angle/1(output1) -> or1/8
  yaw_i/8(output8) -> or8/7
  yaw_i/7(output7) -> or7/7
  yaw_i/6(output6) -> or6/7
  yaw_i/5(output5) -> or5/7
  yaw_i/4(output4) -> or4/7
  yaw_i/3(output3) -> or3/7
  yaw_i/2(output2) -> or2/7
  yaw_i/1(output1) -> or1/7
  yaw_r/8(output8) -> or8/6
  yaw_r/7(output7) -> or7/6
  yaw_r/6(output6) -> or6/6
  yaw_r/5(output5) -> or5/6
  yaw_r/4(output4) -> or4/6
  yaw_r/3(output3) -> or3/6
  yaw_r/2(output2) -> or2/6
  yaw_r/1(output1) -> or1/6
  acc_l/8(output8) -> or8/5
  acc_l/7(output7) -> or7/5
  acc_l/6(output6) -> or6/5
  acc_l/5(output5) -> or5/5
  acc_l/4(output4) -> or4/5
  acc_l/3(output3) -> or3/5
  acc_l/2(output2) -> or2/5
  acc_l/1(output1) -> or1/5
  acc_a/8(output8) -> or8/4
  acc_a/7(output7) -> or7/4
  acc_a/6(output6) -> or6/4
  acc_a/5(output5) -> or5/4
  acc_a/4(output4) -> or4/4
  acc_a/3(output3) -> or3/4
  acc_a/2(output2) -> or2/4
  acc_a/1(output1) -> or1/4
  bre_l/8(output8) -> or8/3
  bre_l/7(output7) -> or7/3
  bre_l/6(output6) -> or6/3
  bre_l/5(output5) -> or5/3
  bre_l/4(output4) -> or4/3
  bre_l/3(output3) -> or3/3
  bre_l/2(output2) -> or2/3
  bre_l/1(output1) -> or1/3
  bre_o_1/8(output8) -> or8/2
  bre_o_1/7(output7) -> or7/2
  bre_o_1/6(output6) -> or6/2
  bre_o_1/5(output5) -> or5/2
  bre_o_1/4(output4) -> or4/2
  bre_o_1/3(output3) -> or3/2
  bre_o_1/2(output2) -> or2/2
  bre_o_1/1(output1) -> or1/2
  bre_o_2/8(output8) -> or8/1
  bre_o_2/7(output7) -> or7/1
  bre_o_2/6(output6) -> or6/1
  bre_o_2/5(output5) -> or5/1
  bre_o_2/4(output4) -> or4/1
  bre_o_2/3(output3) -> or3/1
  bre_o_2/2(output2) -> or2/1
  bre_o_2/1(output1) -> or1/1
  ECU_sig_mux/1 -> output/1

== system 21-E/ECU_can/ECU_speed ==
  v_2R_in : Inport
  v_2L_in : Inport  Port=2
  v_1R_in : Inport  Port=3
  v_1L_in : Inport  Port=4
  Conv{1..8} (8 alike) : DataTypeConversion
  ECU_speed_DLC : Constant  Value=8  OutDataTypeStr=uint8
  ECU_speed_DLC_Out : Terminator
  ECU_speed_ID : Constant  Value=7  OutDataTypeStr=single
  ECU_speed_ID_Out : Terminator
  ECU_speed_mux : Mux  Inputs=8
  or{1..8} (8 alike) : simulink/Logic and Bit Operations/Bitwise Operator  logicop=OR  UseBitMask=off  NumInputPorts=4  BitMask=bin2dec('11011001')  BitMaskRealWorld=Stored Integer
  v_1L : Subsystem
  v_1R : Subsystem
  v_2L : Subsystem
  v_2R : Subsystem
  output : Outport
  wires:
  v_1L_in/1 -> v_1L/1(v_1L)
  v_1R_in/1 -> v_1R/1(v_1R)
  v_2L_in/1 -> v_2L/1(v_2L)
  v_2R_in/1 -> v_2R/1(v_2R)
  ECU_speed_DLC/1 -> ECU_speed_DLC_Out/1
  ECU_speed_ID/1 -> ECU_speed_ID_Out/1
  Conv8/1 -> ECU_speed_mux/8
  or8/1 -> Conv8/1
  Conv7/1 -> ECU_speed_mux/7
  or7/1 -> Conv7/1
  Conv6/1 -> ECU_speed_mux/6
  or6/1 -> Conv6/1
  Conv5/1 -> ECU_speed_mux/5
  or5/1 -> Conv5/1
  Conv4/1 -> ECU_speed_mux/4
  or4/1 -> Conv4/1
  Conv3/1 -> ECU_speed_mux/3
  or3/1 -> Conv3/1
  Conv2/1 -> ECU_speed_mux/2
  or2/1 -> Conv2/1
  Conv1/1 -> ECU_speed_mux/1
  or1/1 -> Conv1/1
  v_1L/8(output8) -> or8/4
  v_1L/7(output7) -> or7/4
  v_1L/6(output6) -> or6/4
  v_1L/5(output5) -> or5/4
  v_1L/4(output4) -> or4/4
  v_1L/3(output3) -> or3/4
  v_1L/2(output2) -> or2/4
  v_1L/1(output1) -> or1/4
  v_1R/8(output8) -> or8/3
  v_1R/7(output7) -> or7/3
  v_1R/6(output6) -> or6/3
  v_1R/5(output5) -> or5/3
  v_1R/4(output4) -> or4/3
  v_1R/3(output3) -> or3/3
  v_1R/2(output2) -> or2/3
  v_1R/1(output1) -> or1/3
  v_2L/8(output8) -> or8/2
  v_2L/7(output7) -> or7/2
  v_2L/6(output6) -> or6/2
  v_2L/5(output5) -> or5/2
  v_2L/4(output4) -> or4/2
  v_2L/3(output3) -> or3/2
  v_2L/2(output2) -> or2/2
  v_2L/1(output1) -> or1/2
  v_2R/8(output8) -> or8/1
  v_2R/7(output7) -> or7/1
  v_2R/6(output6) -> or6/1
  v_2R/5(output5) -> or5/1
  v_2R/4(output4) -> or4/1
  v_2R/3(output3) -> or3/1
  v_2R/2(output2) -> or2/1
  v_2R/1(output1) -> or1/1
  ECU_speed_mux/1 -> output/1

== system 21-E/ECU_can/ECU_tem ==
  Mot_4_in : Inport
  Mot_3_in : Inport  Port=2
  Mot_2_in : Inport  Port=3
  Mot_1_in : Inport  Port=4
  IGBT_4_in : Inport  Port=5
  IGBT_3_in : Inport  Port=6
  IGBT_2_in : Inport  Port=7
  IGBT_1_in : Inport  Port=8
  Conv{1..8} (8 alike) : DataTypeConversion
  ECU_tem_DLC : Constant  Value=8  OutDataTypeStr=uint8
  ECU_tem_DLC_Out : Terminator
  ECU_tem_ID : Constant  Value=6  OutDataTypeStr=single
  ECU_tem_ID_Out : Terminator
  ECU_tem_mux : Mux  Inputs=8
  IGBT_1 : Subsystem
  IGBT_2 : Subsystem
  IGBT_3 : Subsystem
  IGBT_4 : Subsystem
  Mot_1 : Subsystem
  Mot_2 : Subsystem
  Mot_3 : Subsystem
  Mot_4 : Subsystem
  or{1..8} (8 alike) : simulink/Logic and Bit Operations/Bitwise Operator  logicop=OR  UseBitMask=off  NumInputPorts=8  BitMask=bin2dec('11011001')  BitMaskRealWorld=Stored Integer
  output : Outport
  wires:
  IGBT_1_in/1 -> IGBT_1/1(IGBT_1)
  IGBT_2_in/1 -> IGBT_2/1(IGBT_2)
  IGBT_3_in/1 -> IGBT_3/1(IGBT_3)
  IGBT_4_in/1 -> IGBT_4/1(IGBT_4)
  Mot_1_in/1 -> Mot_1/1(Mot_1)
  Mot_2_in/1 -> Mot_2/1(Mot_2)
  Mot_3_in/1 -> Mot_3/1(Mot_3)
  Mot_4_in/1 -> Mot_4/1(Mot_4)
  ECU_tem_DLC/1 -> ECU_tem_DLC_Out/1
  ECU_tem_ID/1 -> ECU_tem_ID_Out/1
  Conv8/1 -> ECU_tem_mux/8
  or8/1 -> Conv8/1
  Conv7/1 -> ECU_tem_mux/7
  or7/1 -> Conv7/1
  Conv6/1 -> ECU_tem_mux/6
  or6/1 -> Conv6/1
  Conv5/1 -> ECU_tem_mux/5
  or5/1 -> Conv5/1
  Conv4/1 -> ECU_tem_mux/4
  or4/1 -> Conv4/1
  Conv3/1 -> ECU_tem_mux/3
  or3/1 -> Conv3/1
  Conv2/1 -> ECU_tem_mux/2
  or2/1 -> Conv2/1
  Conv1/1 -> ECU_tem_mux/1
  or1/1 -> Conv1/1
  IGBT_1/8(output8) -> or8/8
  IGBT_1/7(output7) -> or7/8
  IGBT_1/6(output6) -> or6/8
  IGBT_1/5(output5) -> or5/8
  IGBT_1/4(output4) -> or4/8
  IGBT_1/3(output3) -> or3/8
  IGBT_1/2(output2) -> or2/8
  IGBT_1/1(output1) -> or1/8
  IGBT_2/8(output8) -> or8/7
  IGBT_2/7(output7) -> or7/7
  IGBT_2/6(output6) -> or6/7
  IGBT_2/5(output5) -> or5/7
  IGBT_2/4(output4) -> or4/7
  IGBT_2/3(output3) -> or3/7
  IGBT_2/2(output2) -> or2/7
  IGBT_2/1(output1) -> or1/7
  IGBT_3/8(output8) -> or8/6
  IGBT_3/7(output7) -> or7/6
  IGBT_3/6(output6) -> or6/6
  IGBT_3/5(output5) -> or5/6
  IGBT_3/4(output4) -> or4/6
  IGBT_3/3(output3) -> or3/6
  IGBT_3/2(output2) -> or2/6
  IGBT_3/1(output1) -> or1/6
  IGBT_4/8(output8) -> or8/5
  IGBT_4/7(output7) -> or7/5
  IGBT_4/6(output6) -> or6/5
  IGBT_4/5(output5) -> or5/5
  IGBT_4/4(output4) -> or4/5
  IGBT_4/3(output3) -> or3/5
  IGBT_4/2(output2) -> or2/5
  IGBT_4/1(output1) -> or1/5
  Mot_1/8(output8) -> or8/4
  Mot_1/7(output7) -> or7/4
  Mot_1/6(output6) -> or6/4
  Mot_1/5(output5) -> or5/4
  Mot_1/4(output4) -> or4/4
  Mot_1/3(output3) -> or3/4
  Mot_1/2(output2) -> or2/4
  Mot_1/1(output1) -> or1/4
  Mot_2/8(output8) -> or8/3
  Mot_2/7(output7) -> or7/3
  Mot_2/6(output6) -> or6/3
  Mot_2/5(output5) -> or5/3
  Mot_2/4(output4) -> or4/3
  Mot_2/3(output3) -> or3/3
  Mot_2/2(output2) -> or2/3
  Mot_2/1(output1) -> or1/3
  Mot_3/8(output8) -> or8/2
  Mot_3/7(output7) -> or7/2
  Mot_3/6(output6) -> or6/2
  Mot_3/5(output5) -> or5/2
  Mot_3/4(output4) -> or4/2
  Mot_3/3(output3) -> or3/2
  Mot_3/2(output2) -> or2/2
  Mot_3/1(output1) -> or1/2
  Mot_4/8(output8) -> or8/1
  Mot_4/7(output7) -> or7/1
  Mot_4/6(output6) -> or6/1
  Mot_4/5(output5) -> or5/1
  Mot_4/4(output4) -> or4/1
  Mot_4/3(output3) -> or3/1
  Mot_4/2(output2) -> or2/1
  Mot_4/1(output1) -> or1/1
  ECU_tem_mux/1 -> output/1

== system 21-E/ECU_can/Subsystem ==
  Data Store Read1 : DataStoreRead  DataStoreName=IGBTtemp4
  Data Store Read10 : DataStoreRead  DataStoreName=IGBTtemp3
  Data Store Read2 : DataStoreRead  DataStoreName=temp1
  Data Store Read3 : DataStoreRead  DataStoreName=temp2
  Data Store Read4 : DataStoreRead  DataStoreName=temp3
  Data Store Read5 : DataStoreRead  DataStoreName=temp4
  Data Store Read7 : DataStoreRead  DataStoreName=IGBTtemp1
  Data Store Read9 : DataStoreRead  DataStoreName=IGBTtemp2
  Gain{,1..7} (8 alike) : Gain  Gain=0.1  OutDataTypeStr=double
  Rounding Function{1..8} (8 alike) : Rounding
  tem4 : Outport
  tem3 : Outport  Port=2
  tem2 : Outport  Port=3
  tem1 : Outport  Port=4
  IG4 : Outport  Port=5
  IG3 : Outport  Port=6
  IG2 : Outport  Port=7
  IG1 : Outport  Port=8
  wires:
  Rounding Function3/1 -> IG1/1
  Rounding Function4/1 -> IG2/1
  Rounding Function5/1 -> IG3/1
  Rounding Function1/1 -> IG4/1
  Rounding Function2/1 -> tem1/1
  Rounding Function6/1 -> tem2/1
  Rounding Function7/1 -> tem3/1
  Rounding Function8/1 -> tem4/1
  Data Store Read5/1 -> Gain4/1
  Gain4/1 -> Rounding Function8/1
  Data Store Read4/1 -> Gain2/1
  Gain2/1 -> Rounding Function7/1
  Data Store Read3/1 -> Gain3/1
  Gain3/1 -> Rounding Function6/1
  Data Store Read2/1 -> Gain5/1
  Gain5/1 -> Rounding Function2/1
  Data Store Read1/1 -> Gain6/1
  Gain6/1 -> Rounding Function1/1
  Gain/1 -> Rounding Function3/1
  Data Store Read7/1 -> Gain/1
  Gain1/1 -> Rounding Function4/1
  Data Store Read9/1 -> Gain1/1
  Data Store Read10/1 -> Gain7/1
  Gain7/1 -> Rounding Function5/1
